simulink model "jointsCurrentControl"  (Simulink 10.2)
settings: Solver=FixedStepDiscrete  StartTime=0.0  StopTime=30  FixedStep=Config.tStep  RelTol=1e-3  EnableMultiTasking=on
PostLoadFcn:
  | %% Try to open the static GUI
  | try
  | 
  |     staticGUI = simulinkStaticGUI;
  | 
  | end
InitFcn:
  | %% initialize the simulation
  | cd(fileparts(which(bdroot)));
  | initJointsControl;
  | 
  | %% Try to edit the GUI (the user may have already closed it)
  | try
  | 
  |     %% Update Start Button
  |     set(sl_synch_handles.startButton,'Backgroundcolor',[0.0,1.0,0.0]);
  |     set(sl_synch_handles.startButton,'Enable','on');
  | 
  | end
StartFcn:
  | %% Try to edit the GUI (the user may have already closed it)
  | try
  | 
  |     %% Update Start Button
  |     set(sl_synch_handles.startButton,'Backgroundcolor',[0.8,0.8,0.8]);
  |     set(sl_synch_handles.startButton,'Enable','off');
  | 
  |     %% Update Compile Button
  |     set(sl_synch_handles.compileButton,'Backgroundcolor',[0.8,0.8,0.8]);
  |     set(sl_synch_handles.compileButton,'Enable','off');
  | 
  |     %% Update Exit Button
  |     set(sl_synch_handles.exitButton,'Backgroundcolor',[0.8,0.8,0.8]);
  |     set(sl_synch_handles.exitButton,'Enable','off');
  | 
  | end
StopFcn:
  | %% stop the simulation
  | cd(fileparts(which(bdroot)));
  | stopJointsControl;
  | 
  | %% Try to edit the GUI (the user may have already closed it)
  | try
  | 
  |     %% Update Start Button
  |     if get(sl_synch_handles.checkbox_recompile, 'Value')
  |         set(sl_synch_handles.startButton,'Backgroundcolor',[0.0,1.0,0.0]);
  |         set(sl_synch_handles.startButton,'Enable','on');
  |     end
  | 
  |     %% Update Compile Button
  |     set(sl_synch_handles.compileButton,'Backgroundcolor',[1.0,0.6,0.0]);
  |     set(sl_synch_handles.compileButton,'Enable','on');
  | 
  |     %% Update Exit Button
  |     set(sl_synch_handles.exitButton,'Backgroundcolor',[0.0,1.0,1.0]);
  |     set(sl_synch_handles.exitButton,'Enable','on');
  | 
  | end
undefined symbols (not defined in the file or in its folder): Config, DiscIntNeverNeededParam, k1, k2, k3, Ref, Sat
libraries: WBToolboxLibrary x15
CloseFcn:
  | %% Try to close the GUI (the user might have already closed it)
  | try
  | 
  |     close(simulinkStaticGUI)
  | 
  | end
settings Model: Creator=daniele  LastModifiedBy=giuseppe
settings DataIOCC: LimitDataPoints=on
settings DebuggingCC: UnderspecifiedInitializationDetection=Simplified  MergeDetectMultiDrivingBlocksExec=error  SolverPrmCheckMsg=warning  MultiTaskDSMMsg=warning  MultiTaskCondExecSysMsg=none  FcnCallInpInsideContextMsg=error  AllowSymbolicDim=off  StrictBusMsg=ErrorOnBusTreatedAsVector
settings GRTTargetCC: CombineOutputUpdateFcns=on  GRTInterface=off

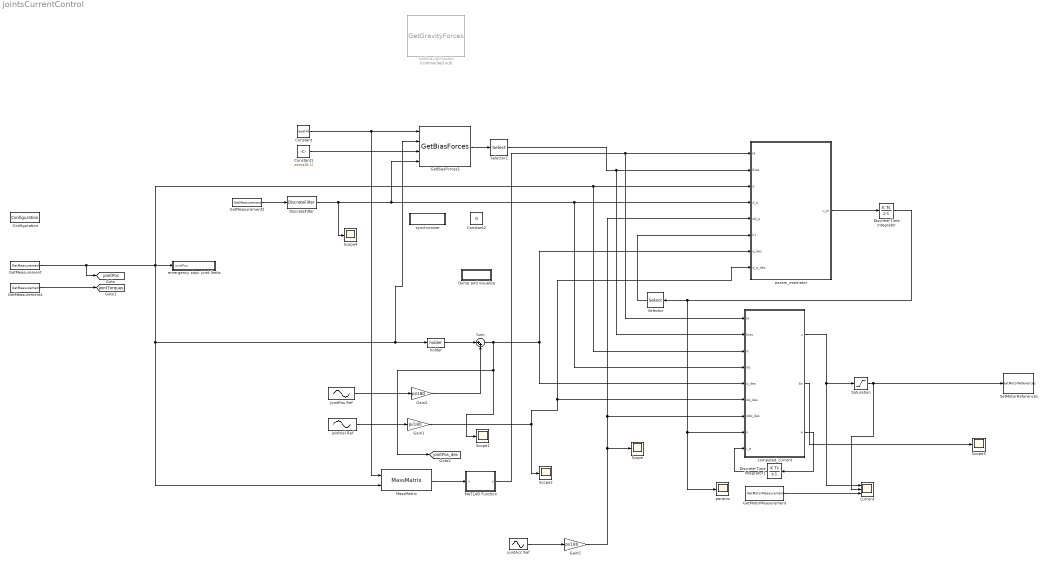
== system jointsCurrentControl ==
  Configuration : WBToolboxLibrary/Utilities/Configuration  ConfigSource=Workspace  ConfigObject='WBTConfigRobot'
      settings: SourceProductName=WholeBodyToolbox
  Constant : Constant  Value=eye(4)
  Constant1 : Constant  Value=zeros(6,1)
  Constant2 : Constant  Value=0
  Discrete-Time Integrator : DiscreteIntegrator  InitialCondition=[k1;k2;k3]  SampleTime=-1  LimitOutput=on  LowerSaturationLimit=[0.01, 0, 0]  ICPrevOutput=DiscIntNeverNeededParam  ICPrevScaledInput=DiscIntNeverNeededParam
  Discrete-Time Integrator1 : DiscreteIntegrator  SampleTime=-1  ICPrevOutput=DiscIntNeverNeededParam  ICPrevScaledInput=DiscIntNeverNeededParam
  DiscreteFilter : WBToolboxLibrary/Utilities/DiscreteFilter  filterType=FirstOrderLowPassFilter  numCoeffs=[0]  denCoeffs=[0]  Fc=1  Ts=0.01  orderMedianFilter=0  initStatus=off  y0=[0]  u0=[0]
      settings: SourceProductName=WholeBodyToolbox
  Dump and visualize : Subsystem
      mask Display: disp('VISUALIZER')
  Gain1 : Gain  Gain=pi/180
  Gain2 : Gain  Gain=pi/180
  Gain5 : Gain  Gain=pi/180
  GetBiasForces1 : WBToolboxLibrary/Model/Dynamics/GetBiasForces
      settings: SourceProductName=WholeBodyToolbox
  GetGravityForces1 : WBToolboxLibrary/Model/Dynamics/GetGravityForces  Commented=on
      settings: SourceProductName=WholeBodyToolbox
  GetMeasurement : WBToolboxLibrary/States/GetMeasurement  measuredType=Joints Position
      settings: SourceProductName=WholeBodyToolbox
  GetMeasurement1 : WBToolboxLibrary/States/GetMeasurement  measuredType=Joints Torque
      settings: SourceProductName=WholeBodyToolbox
  GetMeasurement2 : WBToolboxLibrary/States/GetMeasurement  measuredType=Joints Velocity
      settings: SourceProductName=WholeBodyToolbox
  GetMotorMeasurement : WBToolboxLibrary/States/GetMotorMeasurement  measuredType=Motor Current
      settings: SourceProductName=WholeBodyToolbox
  MATLAB Function : MATLAB Function  TreatAsAtomicUnit=on
  MassMatrix : WBToolboxLibrary/Model/Dynamics/MassMatrix
      settings: SourceProductName=WholeBodyToolbox
  Saturation : Saturate  UpperLimit=3  LowerLimit=-3
  Scope{,1..4} (5 alike) : Scope
  Selector : Selector  InputPortWidth=3  IndexOptions=Index vector (dialog)  Indices=1  OutputSizes=1
  Selector1 : Selector  InputPortWidth=7  IndexOptions=Index vector (dialog)  Indices=7  OutputSizes=1
  SetMotorReferences : WBToolboxLibrary/Actuators/SetMotorReferences  controlType=Current
      settings: SourceProductName=WholeBodyToolbox
  Sum : Sum  Inputs=|++
  computed_current : MATLAB Function  TreatAsAtomicUnit=on
  current : Scope  NumInputPorts=3
  emergency stop: joint limits : Subsystem
      mask Display: disp('EMERGENCY STOP')
  holder : WBToolboxLibrary/Utilities/holder 
      settings: SourceProductName=WholeBodyToolbox
  jointAcc Ref : Sin  Amplitude=-Ref.Amplitude.*(Ref.Frequency.*2.*pi).^2  Frequency=Ref.Frequency.*2.*pi  SampleTime=0
  jointPos Ref : Sin  Amplitude=Ref.Amplitude  Frequency=Ref.Frequency.*2.*pi  SampleTime=0
  jointVel Ref : Sin  Amplitude=Ref.Amplitude.*Ref.Frequency.*2.*pi  Frequency=Ref.Frequency.*2.*pi  Phase=pi/2  SampleTime=0
  param_estimator : MATLAB Function  TreatAsAtomicUnit=on
  params : Scope
  synchronizer : Subsystem
      mask Display: disp('SYNCHRONIZER')
  tag scope: jointPos=global, jointPos_des=global, jointTorques=global
  wires:
  GetMeasurement/1 -> GetBiasForces1/2, holder/1, MassMatrix/2, computed_current/3(q), param_estimator/3(q), emergency stop: joint limits/1(jointPos), [jointPos]
  GetMeasurement1/1 -> [jointTorques]
  Constant/1 -> MassMatrix/1, GetBiasForces1/1
  MassMatrix/1 -> MATLAB Function/1(u)
  param_estimator/1(u_pi) -> Discrete-Time Integrator/1
  Selector/1 -> param_estimator/6(k1)
  Gain2/1 -> Sum/2
  jointPos Ref/1 -> Gain2/1
  Gain1/1 -> param_estimator/8(d_q_des), computed_current/6(dq_des), Scope2/1
  computed_current/1(u) -> Saturation/1, current/1
  MATLAB Function/1(y) -> param_estimator/1(M), computed_current/1(M)
  Selector1/1 -> computed_current/2(bias), param_estimator/2(Bias)
  GetMotorMeasurement/1 -> current/3
  Saturation/1 -> SetMotorReferences/1, current/2
  Discrete-Time Integrator/1 -> Selector/1, params/1, computed_current/8(k)
  holder/1 -> Sum/1
  Gain5/1 -> computed_current/7(ddq_des), param_estimator/5(dd_q), Scope/1
  jointVel Ref/1 -> Gain1/1
  jointAcc Ref/1 -> Gain5/1
  Sum/1 -> [jointPos_des], Scope1/1, computed_current/5(q_des), param_estimator/7(q_des)
  computed_current/2(bo) -> Scope3/1
  computed_current/3(e) -> Discrete-Time Integrator1/1
  Discrete-Time Integrator1/1 -> computed_current/9(i_e)
  GetBiasForces1/1 -> Selector1/1
  Constant1/1 -> GetBiasForces1/3
  GetMeasurement2/1 -> DiscreteFilter/1
  DiscreteFilter/1 -> Scope4/1, GetBiasForces1/4, computed_current/4(dq), param_estimator/4(d_q)

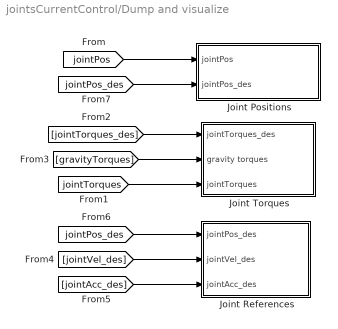
== system jointsCurrentControl/Dump and visualize ==
  Joint Positions : Subsystem
  Joint References : Subsystem
  Joint Torques : Subsystem
  wires:
  [jointTorques] -> Joint Torques/3(jointTorques)
  [gravityTorques] -> Joint Torques/2(gravity torques)
  [jointTorques_des] -> Joint Torques/1(jointTorques_des)
  [jointPos] -> Joint Positions/1(jointPos)
  [jointPos_des] -> Joint References/1(jointPos_des)
  [jointVel_des] -> Joint References/2(jointVel_des)
  [jointAcc_des] -> Joint References/3(jointAcc_des)
  [jointPos_des] -> Joint Positions/2(jointPos_des)

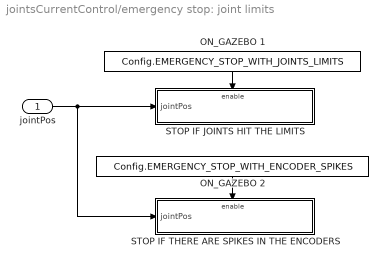
== system jointsCurrentControl/emergency stop: joint limits ==
  jointPos : Inport
  ON_GAZEBO 1 : Constant  Value=Config.EMERGENCY_STOP_WITH_JOINTS_LIMITS
  ON_GAZEBO 2 : Constant  Value=Config.EMERGENCY_STOP_WITH_ENCODER_SPIKES
  STOP IF JOINTS HIT THE LIMITS : Subsystem
  STOP IF THERE ARE SPIKES IN THE ENCODERS : Subsystem
  wires:
  ON_GAZEBO 1/1 -> STOP IF JOINTS HIT THE LIMITS/Enable
  jointPos/1 -> STOP IF THERE ARE SPIKES IN THE ENCODERS/1(jointPos), STOP IF JOINTS HIT THE LIMITS/1(jointPos)
  ON_GAZEBO 2/1 -> STOP IF THERE ARE SPIKES IN THE ENCODERS/Enable

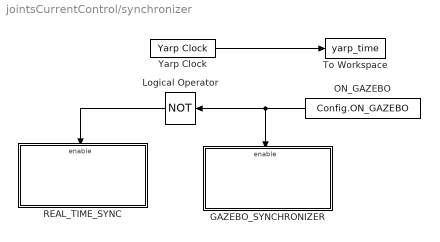
== system jointsCurrentControl/synchronizer ==
  GAZEBO_SYNCHRONIZER : Subsystem
  Logical Operator : Logic  Operator=NOT  AllPortsSameDT=off  OutDataTypeStr=boolean
  "ON_GAZEBO " : Constant  Value=Config.ON_GAZEBO
  REAL_TIME_SYNC : Subsystem
  To Workspace : ToWorkspace  VariableName=yarp_time  SaveFormat=Structure With Time  SampleTime=-1
  Yarp Clock : WBToolboxLibrary/Utilities/Yarp Clock
      settings: SourceProductName=WholeBodyToolbox
  wires:
  Logical Operator/1 -> REAL_TIME_SYNC/Enable
  "ON_GAZEBO "/1 -> GAZEBO_SYNCHRONIZER/Enable, Logical Operator/1
  Yarp Clock/1 -> To Workspace/1

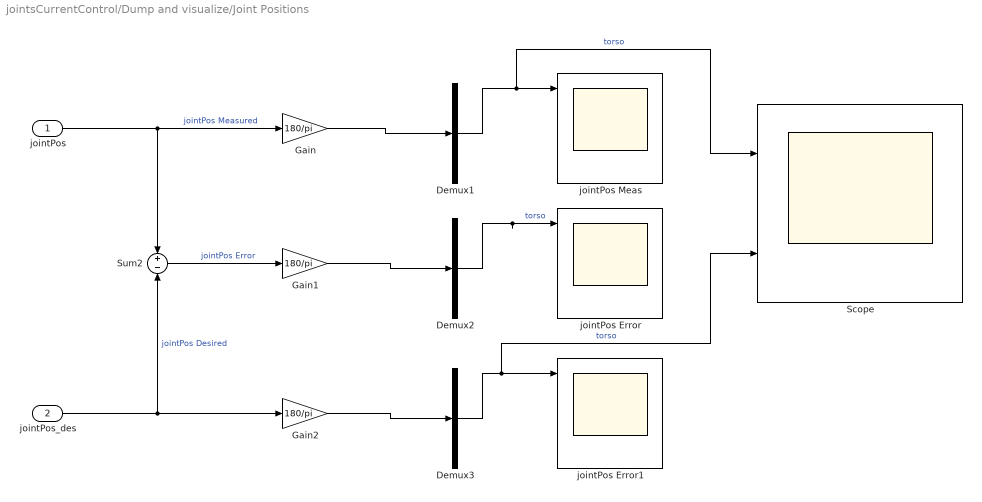
== system jointsCurrentControl/Dump and visualize/Joint Positions ==
  jointPos : Inport
  jointPos_des : Inport  Port=2
  Demux1 : Demux  Outputs=Config.numOfJointsForEachControlboard
  Demux2 : Demux  Outputs=Config.numOfJointsForEachControlboard
  Demux3 : Demux  Outputs=Config.numOfJointsForEachControlboard
  Gain : Gain  Gain=180/pi
  Gain1 : Gain  Gain=180/pi
  Gain2 : Gain  Gain=180/pi
  Scope : Scope  NumInputPorts=2
  Sum2 : Sum  Inputs=+|-
  jointPos Error : Scope  NumInputPorts=5
  jointPos Error1 : Scope  NumInputPorts=5
  jointPos Meas : Scope  NumInputPorts=5
  wires:
  jointPos/1 -> Sum2/1, Gain/1  "jointPos Measured"
  Demux1/1 -> Scope/1, jointPos Meas/1  "torso"
  Demux2/1 -> jointPos Error/1  "torso"
  Sum2/1 -> Gain1/1  "jointPos Error"
  Demux3/1 -> Scope/2, jointPos Error1/1  "torso"
  jointPos_des/1 -> Gain2/1, Sum2/2  "jointPos Desired"
  Gain/1 -> Demux1/1
  Gain1/1 -> Demux2/1
  Gain2/1 -> Demux3/1

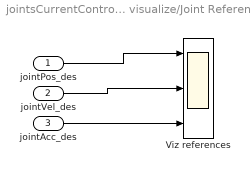
== system jointsCurrentControl/Dump and visualize/Joint References ==
  jointPos_des : Inport
  jointVel_des : Inport  Port=2
  jointAcc_des : Inport  Port=3
  Viz references : Scope  NumInputPorts=3
  wires:
  jointAcc_des/1 -> Viz references/3
  jointVel_des/1 -> Viz references/2
  jointPos_des/1 -> Viz references/1

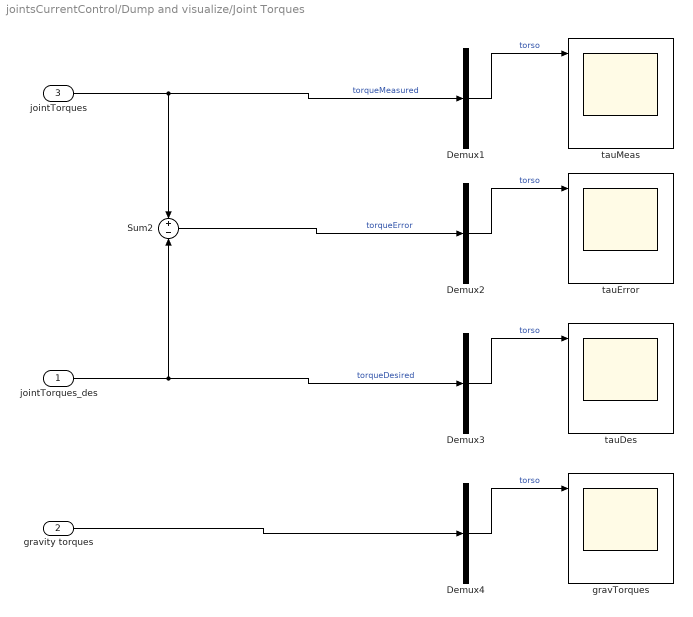
== system jointsCurrentControl/Dump and visualize/Joint Torques ==
  jointTorques_des : Inport
  gravity torques : Inport  Port=2
  jointTorques : Inport  Port=3
  Demux{1..4} (4 alike) : Demux  Outputs=Config.numOfJointsForEachControlboard
  Sum2 : Sum  Inputs=+|-
  gravTorques : Scope  NumInputPorts=5
  tauDes : Scope  NumInputPorts=5
  tauError : Scope  NumInputPorts=5
  tauMeas : Scope  NumInputPorts=5
  wires:
  gravity torques/1 -> Demux4/1
  jointTorques/1 -> Demux1/1, Sum2/1  "torqueMeasured"
  Demux1/1 -> tauMeas/1  "torso"
  ? -> tauMeas/2  "left_arm"
  ? -> tauMeas/4  "left_leg"
  ? -> tauMeas/3  "right_arm"
  ? -> tauMeas/5  "right_leg"
  Demux2/1 -> tauError/1  "torso"
  ? -> tauError/2  "left_arm"
  ? -> tauError/4  "left_leg"
  ? -> tauError/3  "right_arm"
  ? -> tauError/5  "right_leg"
  Sum2/1 -> Demux2/1  "torqueError"
  Demux3/1 -> tauDes/1  "torso"
  ? -> tauDes/2  "left_arm"
  ? -> tauDes/4  "left_leg"
  ? -> tauDes/3  "right_arm"
  jointTorques_des/1 -> Demux3/1, Sum2/2  "torqueDesired"
  ? -> tauDes/5  "right_leg"
  Demux4/1 -> gravTorques/1  "torso"
  ? -> gravTorques/2  "left_arm"
  ? -> gravTorques/4  "left_leg"
  ? -> gravTorques/3  "right_arm"
  ? -> gravTorques/5  "right_leg"

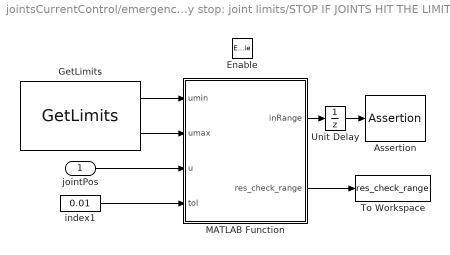
== system jointsCurrentControl/emergency stop: joint limits/STOP IF JOINTS HIT THE LIMITS ==
  jointPos : Inport
  Enable : EnablePort
  Assertion : Assertion
  GetLimits : WBToolboxLibrary/States/GetLimits  limitsSource=ControlBoard  limitsType=Position
      settings: SourceProductName=WholeBodyToolbox
  MATLAB Function : MATLAB Function  TreatAsAtomicUnit=on
  To Workspace : ToWorkspace  VariableName=res_check_range  SaveFormat=Structure With Time  SampleTime=Config.tStep
  Unit Delay : UnitDelay  InitialCondition=1  SampleTime=Config.tStep  HasFrameUpgradeWarning=on
  index1 : Constant  Value=0.01  VectorParams1D=off
  wires:
  jointPos/1 -> MATLAB Function/3(u)
  MATLAB Function/1(inRange) -> Unit Delay/1
  index1/1 -> MATLAB Function/4(tol)
  MATLAB Function/2(res_check_range) -> To Workspace/1
  Unit Delay/1 -> Assertion/1
  GetLimits/1 -> MATLAB Function/1(umin)
  GetLimits/2 -> MATLAB Function/2(umax)

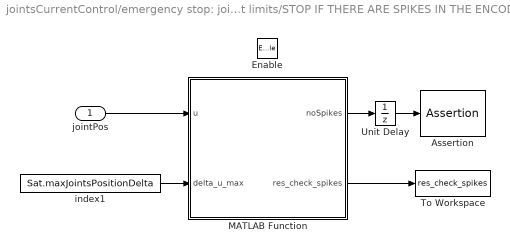
== system jointsCurrentControl/emergency stop: joint limits/STOP IF THERE ARE SPIKES IN THE ENCODERS ==
  jointPos : Inport
  Enable : EnablePort
  Assertion : Assertion
  MATLAB Function : MATLAB Function  TreatAsAtomicUnit=on
  To Workspace : ToWorkspace  VariableName=res_check_spikes  SaveFormat=Structure With Time  SampleTime=Config.tStep
  Unit Delay : UnitDelay  InitialCondition=1  SampleTime=Config.tStep  HasFrameUpgradeWarning=on
  index1 : Constant  Value=Sat.maxJointsPositionDelta  VectorParams1D=off
  wires:
  jointPos/1 -> MATLAB Function/1(u)
  MATLAB Function/1(noSpikes) -> Unit Delay/1
  index1/1 -> MATLAB Function/2(delta_u_max)
  MATLAB Function/2(res_check_spikes) -> To Workspace/1
  Unit Delay/1 -> Assertion/1

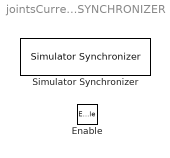
== system jointsCurrentControl/synchronizer/GAZEBO_SYNCHRONIZER ==
  Enable : EnablePort
  Simulator Synchronizer : WBToolboxLibrary/Utilities/Simulator Synchronizer  period=Config.tStep  serverPortName='/clock/rpc'  clientPortName='/WBT_synchronizer/rpc:o'
      settings: SourceProductName=WholeBodyToolbox

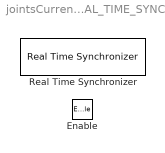
== system jointsCurrentControl/synchronizer/REAL_TIME_SYNC ==
  Enable : EnablePort
  Real Time Synchronizer : WBToolboxLibrary/Utilities/Real Time Synchronizer  period=Config.tStep
      settings: SourceProductName=WholeBodyToolbox

== matlab function computed_current ==
  data: M input double; u output double; bias input double; q input double; dq input double; q_des input double; dq_des input double; ddq_des input double; k input double; bo output double; e output double; i_e input double
function [u, bo, e]= ctrl_current(M, bias, q, dq, q_des, dq_des, ddq_des, k, i_e)
k1 = k(1);
k2 = k(2);
k3 = k(3);
Kp = 100;
Kv = 2 * sqrt(Kp)/10;
KI = 0;
e = q_des - q;
de = dq_des - dq;
u = diag(k1) * (M * (ddq_des + Kp * e + Kv * de + KI * i_e) + 1 * bias) + diag(k2) * dq + diag(k3) * tanh(100 * dq);
bo = M * (ddq_des + Kp * e + Kv * de) + 1 * bias;

== matlab function param_estimator ==
  data: M input double; u_pi output double; Bias input double; q input double; d_q input double; dd_q input double; k1 input double; q_des input double; d_q_des input double
function u_pi = ctrl_param(M, Bias, q, d_q, dd_q, k1, q_des, d_q_des)
Y = [ diag(M * dd_q + Bias), diag(d_q), diag(tanh(100 * d_q))]
R = 100 * eye(size(Y,2));
siz = length(Bias);
B = [zeros(siz); eye(siz)];
% P = 1 * eye(2 * siz);
P = diag([1, 2]);
e = q_des - q;
d_e = d_q_des - d_q;
u_pi = R \ (Y' * (inv(diag(k1) * M))' * B' * P * [e; d_e]);

== matlab function MATLAB Function ==
  data: u input double; y output double
function y = fcn(u)
y = u(7:end, 7:end);

== matlab function emergency stop: joint limits/STOP IF THERE ARE SPIKES IN THE ENCODERS/MATLAB Function ==
  data: u input double; delta_u_max input double; noSpikes output double; res_check_spikes output double
function [noSpikes, res_check_spikes] = checkInputSpikesFCN(u, delta_u_max)

     [noSpikes, res_check_spikes] = wbc.checkInputSpikes(u, delta_u_max);
end

== matlab function emergency stop: joint limits/STOP IF JOINTS HIT THE LIMITS/MATLAB Function ==
  data: umin input double; umax input double; u input double; inRange output double; tol input double; res_check_range output double
function [inRange, res_check_range] = checkInputRangeFCN(umin, umax, u, tol)

     [inRange, res_check_range] = wbc.checkInputRange(umin, umax, u, tol);
end
